simulink model "simulink3"  (R2020b)
settings: Solver=VariableStepAuto  StartTime=0.0  StopTime=50  RelTol=1e-3
settings Model: Creator=akku  LastModifiedBy=akku

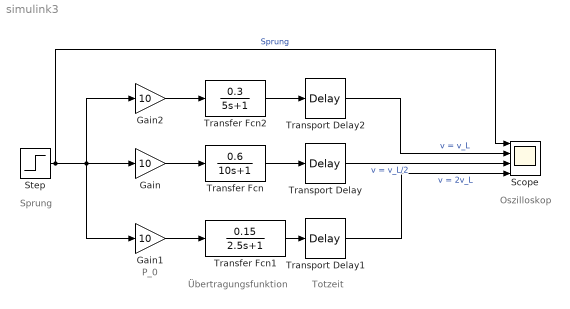
== system simulink3 ==
  note: Oszilloskop
  note: Totzeit
  note: Übertragungsfunktion
  note: P_0
  note: Sprung
  Gain : Gain  Gain=10
  Gain1 : Gain  Gain=10
  Gain2 : Gain  Gain=10
  Scope : Scope  NumInputPorts=4
  Step : Step  Time=0  SampleTime=0
  Transfer Fcn : TransferFcn  Numerator=[0.6]  Denominator=[10 1]
  Transfer Fcn1 : TransferFcn  Numerator=[0.15]  Denominator=[2.5 1]
  Transfer Fcn2 : TransferFcn  Numerator=[0.3]  Denominator=[5 1]
  Transport Delay : TransportDelay
  Transport Delay1 : TransportDelay
  Transport Delay2 : TransportDelay
  wires:
  Step/1 -> Scope/1, Gain1/1, Gain2/1, Gain/1  "Sprung"
  Transport Delay/1 -> Scope/3  "v = v_L/2"
  Gain/1 -> Transfer Fcn/1
  Transport Delay2/1 -> Scope/2  "v = v_L"
  Transfer Fcn/1 -> Transport Delay/1
  Gain1/1 -> Transfer Fcn1/1
  Gain2/1 -> Transfer Fcn2/1
  Transfer Fcn1/1 -> Transport Delay1/1
  Transfer Fcn2/1 -> Transport Delay2/1
  Transport Delay1/1 -> Scope/4  "v = 2v_L"
